simulink model "Variable_order_model"  (R2018b)
settings: Solver=VariableStepAuto  StartTime=0.0  StopTime=2000.0  RelTol=1e-3
undefined symbols (not defined in the file): a0, a1, alpha0, alpha1, k, rho, specificHeat
libraries: voderiv x3
settings Model: Creator=user  LastModifiedBy=user
settings SFSimCC: SimUseLocalCustomCode=off
settings RTWCC: RTWUseLocalCustomCode=off
settings CodeAppCC: StateflowObjectComments=on

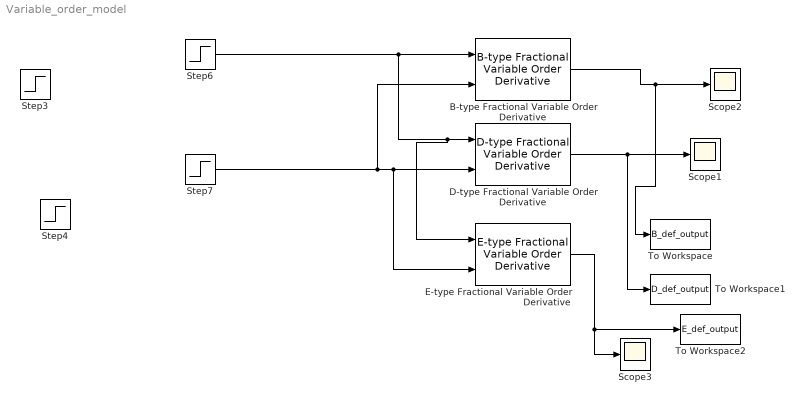
== system Variable_order_model ==
  B-type Fractional Variable Order Derivative : voderiv/B-type Fractional Variable Order Derivative  N=1  Nbuf=20000  Ts=0.1
  D-type Fractional Variable Order Derivative : voderiv/D-type Fractional Variable Order Derivative  N=1  Nbuf=20000  Ts=0.1
  E-type Fractional Variable Order Derivative : voderiv/E-type Fractional Variable Order Derivative  N=1  Nbuf=2000  Ts=1
  Scope1 : Scope
  Scope2 : Scope
  Scope3 : Scope
  Step3 : Step  Time=500  Before=500/sqrt(10)*(9.9878e-5)  After=500/sqrt(10)*(6.2051e-5)  SampleTime=0
  Step4 : Step  Time=500  Before=-0.5  After=-1.2686/2  SampleTime=0
  Step6 : Step  Time=1000  Before=500/(sqrt(rho*specificHeat/k)/a0)  After=500/(sqrt(rho*specificHeat/k)/a1)  SampleTime=0
  Step7 : Step  Time=1000  Before=-alpha0/2  After=-alpha1/2  SampleTime=0
  To Workspace : ToWorkspace  VariableName=B_def_output  SampleTime=0.025
      settings: Decimation=10
  To Workspace1 : ToWorkspace  VariableName=D_def_output  SampleTime=0.025
      settings: Decimation=10
  To Workspace2 : ToWorkspace  VariableName=E_def_output  SampleTime=0.025
      settings: Decimation=10
  wires:
  B-type Fractional Variable Order Derivative/1 -> To Workspace/1, Scope2/1
  D-type Fractional Variable Order Derivative/1 -> To Workspace1/1, Scope1/1
  Step7/1 -> B-type Fractional Variable Order Derivative/2, E-type Fractional Variable Order Derivative/2, D-type Fractional Variable Order Derivative/2
  Step6/1 -> E-type Fractional Variable Order Derivative/1, D-type Fractional Variable Order Derivative/1, B-type Fractional Variable Order Derivative/1
  E-type Fractional Variable Order Derivative/1 -> To Workspace2/1, Scope3/1
